simulink model "GVCU_HIL"  (R2026a)
settings: Solver=ode3  StartTime=0  StopTime=2474  FixedStep=0.0002
model workspace (MAT data in the model file):
  CANoelibParameters : object (value not decoded)
values from neighbouring files (symbols this model uses):
  acc_pedal_data = pedal_data.accelerator_pedal_position_t0    [Vehicle_Simulink_init.m]
  acc_pedal_time = pedal_data.t0    [Vehicle_Simulink_init.m]
  brk_pedal_data = brake_pedal_data.shared_brakes_drvrBrkPedlPerc_t0    [Vehicle_Simulink_init.m]
  brk_pedal_time = brake_pedal_data.t0    [Vehicle_Simulink_init.m]
  cycle_len = zeros(1, num_cycles)    [Vehicle_Simulink_init.m]
  cycle_speed_matrix = zeros(max_cycle_len, num_cycles)    [Vehicle_Simulink_init.m]
  cycle_time_matrix = zeros(max_cycle_len, num_cycles)    [Vehicle_Simulink_init.m]
  veh_speed_data = speed_data.shared_dynamicsVso_vehVelLgt_t0    [Vehicle_Simulink_init.m]
  veh_speed_time = speed_data.t0    [Vehicle_Simulink_init.m]
undefined symbols (not defined in the file or in its folder): Active, AuxActive, bat, environment, FL_prs_voltage, FR_prs_voltage, pos, RL_prs_voltage, RR_prs_voltage, tir, veh, VGetRawValueFlag, Voltage, VT2816_1_Ch1, VT2816_1_Ch2, VT2816_1_Ch3, VT2816_1_Ch4, VT2816_3_Ch13, VT2816_3_Ch14, VT7101_1_Out2, VT7820_2_Channel1, VT7820_2_Channel2, VT7820_2_Channel3, VT7820_2_Channel4, VTS
libraries: canoelib x144, autolibsharedcoupling x21, autolibcoupling x9, autolibshared x5, simulink_extras x4, simulink x4, slpidlib x3, autolibshareddiff x3, autolibutils x1, autolibdatasheetbattery x1, autolibmappedmotor x1, sl_discontinuities x1
(part 4 of 9)

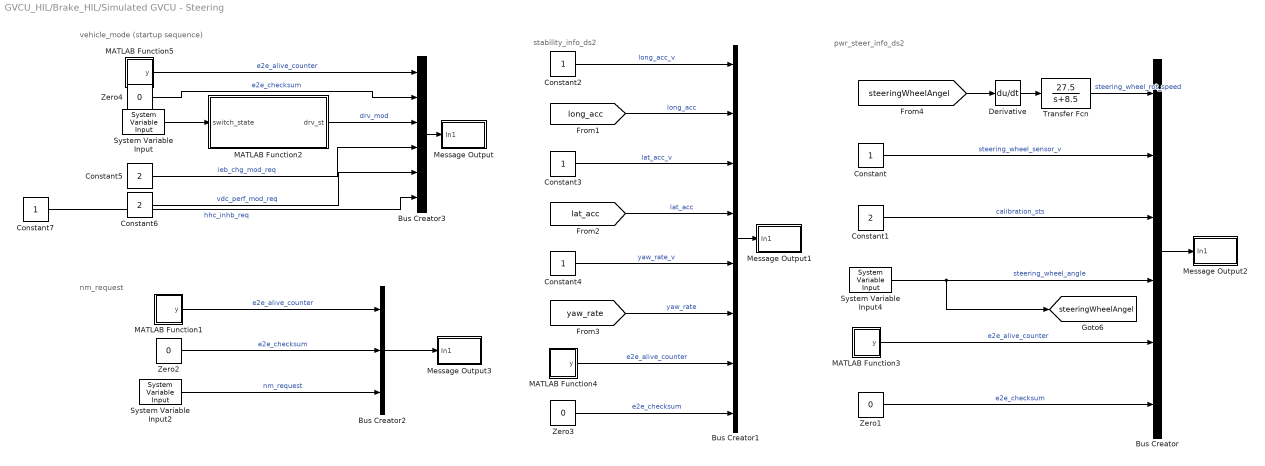
== system GVCU_HIL/Brake_HIL/Simulated GVCU - Steering  ==
  note: pwr_steer_info_ds2
  note: stability_info_ds2
  note: vehicle_mode (startup sequence)
  note: nm_request
  Bus Creator : BusCreator  Inputs=6
  Bus Creator1 : BusCreator  Inputs=8
  Bus Creator2 : BusCreator  Inputs=3
  Bus Creator3 : BusCreator  Inputs=6
  Constant{,2..4,7} (5 alike) : Constant
  Constant1 : Constant  Value=2
  Constant5 : Constant  Value=2
  Constant6 : Constant  Value=2
  Derivative : Derivative
  MATLAB Function1 : MATLAB Function  TreatAsAtomicUnit=on
  MATLAB Function2 : MATLAB Function  TreatAsAtomicUnit=on
  MATLAB Function3 : MATLAB Function  TreatAsAtomicUnit=on
  MATLAB Function4 : MATLAB Function  TreatAsAtomicUnit=on
  MATLAB Function5 : MATLAB Function  TreatAsAtomicUnit=on
  Message Output : Subsystem  AncestorBlock=canoelib/CANoe I//O/Message Output  mask(Signal Output Module){dbName=IEB_DBC_V32, nodeName=GVCU, msgName=vehicle_mode, inputType=Bus Signal, rawValue=Default}
      mask prompts: dbName "Database name"; nodeName "Node name"; msgName "Message name"; inputType "Input type"; rawValue "Raw value"
      mask help: Output module for all signals of a databasemessage provided by the CANoe interaction layer. Double click the block for configuration.
      settings: AttributesFormatString=%<msgName>  CopyFcn=set_param(gcb, 'AttributesFormatString', '%<msgName>');  OpenFcn=MessageOutputBlock
      mask Help: For detailed information please refer to the CANoe online help 'MATLAB Integration Package » CANoe I/O Library'.
      mask TypeOptions inputType: Vector | Bus Signal
      mask TypeOptions rawValue: Default | Physical value | Raw value
      mask Display:
      | image(imread('MatlabBlock.png'))
      | disp('CANoe')
  Message Output1 : Subsystem  AncestorBlock=canoelib/CANoe I//O/Message Output  mask(Signal Output Module){dbName=IEB_DBC_V32, nodeName=GVCU, msgName=stability_info_ds2, inputType=Bus Signal, rawValue=Default}
      mask prompts: dbName "Database name"; nodeName "Node name"; msgName "Message name"; inputType "Input type"; rawValue "Raw value"
      mask help: Output module for all signals of a databasemessage provided by the CANoe interaction layer. Double click the block for configuration.
      settings: AttributesFormatString=%<msgName>  CopyFcn=set_param(gcb, 'AttributesFormatString', '%<msgName>');  OpenFcn=MessageOutputBlock
      mask Help: For detailed information please refer to the CANoe online help 'MATLAB Integration Package » CANoe I/O Library'.
      mask TypeOptions inputType: Vector | Bus Signal
      mask TypeOptions rawValue: Default | Physical value | Raw value
      mask Display:
      | image(imread('MatlabBlock.png'))
      | disp('CANoe')
  Message Output2 : Subsystem  AncestorBlock=canoelib/CANoe I//O/Message Output  mask(Signal Output Module){dbName=IEB_DBC_V32, nodeName=GVCU, msgName=pwr_steer_info_ds2, inputType=Bus Signal, rawValue=Default}
      mask prompts: dbName "Database name"; nodeName "Node name"; msgName "Message name"; inputType "Input type"; rawValue "Raw value"
      mask help: Output module for all signals of a databasemessage provided by the CANoe interaction layer. Double click the block for configuration.
      settings: AttributesFormatString=%<msgName>  CopyFcn=set_param(gcb, 'AttributesFormatString', '%<msgName>');  OpenFcn=MessageOutputBlock
      mask Help: For detailed information please refer to the CANoe online help 'MATLAB Integration Package » CANoe I/O Library'.
      mask TypeOptions inputType: Vector | Bus Signal
      mask TypeOptions rawValue: Default | Physical value | Raw value
      mask Display:
      | image(imread('MatlabBlock.png'))
      | disp('CANoe')
  Message Output3 : Subsystem  AncestorBlock=canoelib/CANoe I//O/Message Output  mask(Signal Output Module){dbName=IEB_DBC_V32, nodeName=GVCU, msgName=nm_request_gvcu_ds2, inputType=Bus Signal, rawValue=Default}
      mask prompts: dbName "Database name"; nodeName "Node name"; msgName "Message name"; inputType "Input type"; rawValue "Raw value"
      mask help: Output module for all signals of a databasemessage provided by the CANoe interaction layer. Double click the block for configuration.
      settings: AttributesFormatString=%<msgName>  CopyFcn=set_param(gcb, 'AttributesFormatString', '%<msgName>');  OpenFcn=MessageOutputBlock
      mask Help: For detailed information please refer to the CANoe online help 'MATLAB Integration Package » CANoe I/O Library'.
      mask TypeOptions inputType: Vector | Bus Signal
      mask TypeOptions rawValue: Default | Physical value | Raw value
      mask Display:
      | image(imread('MatlabBlock.png'))
      | disp('CANoe')
  System Variable Input : canoelib/CANoe I//O/System Variable Input  nsName=ABS_TEST  sysVarName=Acceleration  arrayIndex=-1  editSampleTime=0  rawValue=Default  dataType=Default  dataTypeDB=int32  hasEncoding=off  dataTypeCANoe=Get from CANoe
      settings: AttributesFormatString=%<nsName>::%<sysVarName>  SourceProductName=Vector CANoe
  System Variable Input2 : canoelib/CANoe I//O/System Variable Input  nsName=ABS_TEST  sysVarName=NM_request_Model  arrayIndex=-1  editSampleTime=0  rawValue=Default  dataType=Default  dataTypeDB=uint32  hasEncoding=off  dataTypeCANoe=Get from CANoe
      settings: AttributesFormatString=%<nsName>::%<sysVarName>  SourceProductName=Vector CANoe
  System Variable Input4 : canoelib/CANoe I//O/System Variable Input  nsName=ABS_TEST  sysVarName=steering_ang  arrayIndex=-1  editSampleTime=0  rawValue=Default  dataType=Default  dataTypeDB=double  hasEncoding=off  dataTypeCANoe=Get from CANoe
      settings: AttributesFormatString=%<nsName>::%<sysVarName>  SourceProductName=Vector CANoe
  Transfer Fcn : TransferFcn  Numerator=[27.5]  Denominator=[1 8.5]
  Zero{1..4} (4 alike) : Constant  Value=0  OutDataTypeStr=Inherit: Inherit via back propagation
  tag scope: steeringWheelAngel=global
  wires:
  Transfer Fcn/1 -> Bus Creator/1  "steering_wheel_rot_speed"
  Derivative/1 -> Transfer Fcn/1
  [steeringWheelAngel] -> Derivative/1
  MATLAB Function1/1(y) -> Bus Creator2/1  "e2e_alive_counter"
  MATLAB Function4/1(y) -> Bus Creator1/7  "e2e_alive_counter"
  MATLAB Function5/1(y) -> Bus Creator3/1  "e2e_alive_counter"
  MATLAB Function3/1(y) -> Bus Creator/5  "e2e_alive_counter"
  Bus Creator3/1 -> Message Output/1(In1)
  Zero4/1 -> Bus Creator3/2  "e2e_checksum"
  Bus Creator2/1 -> Message Output3/1(In1)
  Zero2/1 -> Bus Creator2/2  "e2e_checksum"
  System Variable Input2/1 -> Bus Creator2/3  "nm_request"
  Constant6/1 -> Bus Creator3/5  "vdc_perf_mod_req"
  Constant5/1 -> Bus Creator3/4  "ieb_chg_mod_req"
  System Variable Input/1 -> MATLAB Function2/1(switch_state)
  MATLAB Function2/1(drv_st) -> Bus Creator3/3  "drv_mod"
  Bus Creator1/1 -> Message Output1/1(In1)
  [yaw_rate] -> Bus Creator1/6  "yaw_rate"
  [long_acc] -> Bus Creator1/2  "long_acc"
  [lat_acc] -> Bus Creator1/4  "lat_acc"
  Zero3/1 -> Bus Creator1/8  "e2e_checksum"
  Constant4/1 -> Bus Creator1/5  "yaw_rate_v"
  Constant3/1 -> Bus Creator1/3  "lat_acc_v"
  Constant2/1 -> Bus Creator1/1  "long_acc_v"
  Bus Creator/1 -> Message Output2/1(In1)
  Zero1/1 -> Bus Creator/6  "e2e_checksum"
  System Variable Input4/1 -> Bus Creator/4, [steeringWheelAngel]  "steering_wheel_angle"
  Constant1/1 -> Bus Creator/3  "calibration_sts"
  Constant7/1 -> Bus Creator3/6  "hhc_inhb_req"
  Constant/1 -> Bus Creator/2  "steering_wheel_sensor_v"

== system GVCU_HIL/Clutch handling/Offset prs setting ==
  prs_to_voltage : Inport
  Offset setting : Constant  Value=0
  Step : Step  Time=0.2  SampleTime=0
  Switch : Switch  Criteria=u2 > Threshold  SaturateOnIntegerOverflow=off  InputSameDT=off
  Out1 : Outport
  wires:
  Step/1 -> Switch/2
  Offset setting/1 -> Switch/3
  Switch/1 -> Out1/1
  prs_to_voltage/1 -> Switch/1

== system GVCU_HIL/Clutch handling/Offset prs setting1 ==
  prs_to_voltage : Inport
  Offset setting : Constant  Value=0
  Step : Step  Time=0.2  SampleTime=0
  Switch : Switch  Criteria=u2 > Threshold  SaturateOnIntegerOverflow=off  InputSameDT=off
  Out1 : Outport
  wires:
  Step/1 -> Switch/2
  Offset setting/1 -> Switch/3
  Switch/1 -> Out1/1
  prs_to_voltage/1 -> Switch/1

== system GVCU_HIL/Clutch handling/Offset prs setting2 ==
  prs_to_voltage : Inport
  Offset setting : Constant  Value=0
  Step : Step  Time=0.2  SampleTime=0
  Switch : Switch  Criteria=u2 > Threshold  SaturateOnIntegerOverflow=off  InputSameDT=off
  Out1 : Outport
  wires:
  Step/1 -> Switch/2
  Offset setting/1 -> Switch/3
  Switch/1 -> Out1/1
  prs_to_voltage/1 -> Switch/1

== system GVCU_HIL/Clutch handling/Offset prs setting3 ==
  prs_to_voltage : Inport
  Offset setting : Constant  Value=0
  Step : Step  Time=0.2  SampleTime=0
  Switch : Switch  Criteria=u2 > Threshold  SaturateOnIntegerOverflow=off  InputSameDT=off
  Out1 : Outport
  wires:
  Step/1 -> Switch/2
  Offset setting/1 -> Switch/3
  Switch/1 -> Out1/1
  prs_to_voltage/1 -> Switch/1

== system GVCU_HIL/Clutch handling/Offset_substraction ==
  prs_to_voltage : Inport
  MATLAB Function : MATLAB Function  TreatAsAtomicUnit=on
  Signal Input : canoelib/CANoe I//O/Signal Input  dbName=dynamic_systems1_bus  nodeName=GVCU  msgName=vehicle_status_ds1  sigName=drv_mod  editSampleTime=0  rawValue=Default  dataType=Default  dataTypeDB=uint8  hasEncoding=off
      settings: AttributesFormatString=%<sigName>  SourceProductName=Vector CANoe
  y : Outport
  wires:
  Signal Input/1 -> MATLAB Function/1(drvMode)
  MATLAB Function/1(y) -> y/1
  prs_to_voltage/1 -> MATLAB Function/2(pPa)

== system GVCU_HIL/Clutch handling/cur_to_prs ==
  note: Dither filtering
  note: breakpoints out of real measurement
  In1 : Inport
  1-D Lookup Table2 : Lookup_n-D  NumberOfTableDimensions=1  BreakpointsForDimension1=[14.52 16.75 17.32 24.99]  Table=[1.02 3.38 3.68 11.09]  InternalRulePriority=Speed  RndMeth=Simplest
  1-D Lookup Table9 : Lookup_n-D  NumberOfTableDimensions=1  BreakpointsForDimension1=[0.584 0.786 0.882 0.992]  Table=[14.62 19.62 22.19 24.95]  InternalRulePriority=Speed  RndMeth=Simplest
  Constant : Constant  Value=0
  Gain : Gain  Gain=100000
  Switch2 : Switch  Criteria=u2 > Threshold  Threshold=0.1  SaturateOnIntegerOverflow=off  InputSameDT=off
  Transfer Fcn : TransferFcn  Denominator=[1 1]
  Out1 : Outport
  wires:
  Switch2/1 -> Out1/1
  1-D Lookup Table9/1 -> 1-D Lookup Table2/1  "cluCMD [%]"
  In1/1 -> Transfer Fcn/1  "solnDrvrCur [A]"
  Constant/1 -> Switch2/3
  1-D Lookup Table2/1 -> Gain/1  "whlCluPress [bar]"
  Gain/1 -> Switch2/1  "[Pa]"
  Transfer Fcn/1 -> 1-D Lookup Table9/1, Switch2/2

== system GVCU_HIL/Clutch handling/cur_to_prs1 ==
  note: Dither filtering
  note: breakpoints out of real measurement
  In1 : Inport
  1-D Lookup Table2 : Lookup_n-D  NumberOfTableDimensions=1  BreakpointsForDimension1=[14.52 16.75 17.32 24.99]  Table=[1.02 3.38 3.68 11.09]  InternalRulePriority=Speed  RndMeth=Simplest
  1-D Lookup Table9 : Lookup_n-D  NumberOfTableDimensions=1  BreakpointsForDimension1=[0.584 0.786 0.882 0.992]  Table=[14.62 19.62 22.19 24.95]  InternalRulePriority=Speed  RndMeth=Simplest
  Constant : Constant  Value=0
  Gain : Gain  Gain=100000
  Switch2 : Switch  Criteria=u2 > Threshold  Threshold=0.1  SaturateOnIntegerOverflow=off  InputSameDT=off
  Transfer Fcn : TransferFcn  Denominator=[1 1]
  Out1 : Outport
  wires:
  Switch2/1 -> Out1/1
  1-D Lookup Table9/1 -> 1-D Lookup Table2/1  "cluCMD [%]"
  In1/1 -> Transfer Fcn/1  "solnDrvrCur [A]"
  Constant/1 -> Switch2/3
  1-D Lookup Table2/1 -> Gain/1  "whlCluPress [bar]"
  Gain/1 -> Switch2/1  "[Pa]"
  Transfer Fcn/1 -> 1-D Lookup Table9/1, Switch2/2

== system GVCU_HIL/Clutch handling/cur_to_prs2 ==
  note: Dither filtering
  note: breakpoints out of real measurement
  In1 : Inport
  1-D Lookup Table2 : Lookup_n-D  NumberOfTableDimensions=1  BreakpointsForDimension1=[14.52 16.75 17.32 24.99]  Table=[1.02 3.38 3.68 11.09]  InternalRulePriority=Speed  RndMeth=Simplest
  1-D Lookup Table9 : Lookup_n-D  NumberOfTableDimensions=1  BreakpointsForDimension1=[0.584 0.786 0.882 0.992]  Table=[14.62 19.62 22.19 24.95]  InternalRulePriority=Speed  RndMeth=Simplest
  Constant : Constant  Value=0
  Gain : Gain  Gain=100000
  Switch2 : Switch  Criteria=u2 > Threshold  Threshold=0.1  SaturateOnIntegerOverflow=off  InputSameDT=off
  Transfer Fcn : TransferFcn  Denominator=[1 1]
  Out1 : Outport
  wires:
  Switch2/1 -> Out1/1
  1-D Lookup Table9/1 -> 1-D Lookup Table2/1  "cluCMD [%]"
  In1/1 -> Transfer Fcn/1  "solnDrvrCur [A]"
  Constant/1 -> Switch2/3
  1-D Lookup Table2/1 -> Gain/1  "whlCluPress [bar]"
  Gain/1 -> Switch2/1  "[Pa]"
  Transfer Fcn/1 -> 1-D Lookup Table9/1, Switch2/2

== system GVCU_HIL/Clutch handling/cur_to_prs3 ==
  note: Dither filtering
  note: breakpoints out of real measurement
  In1 : Inport
  1-D Lookup Table2 : Lookup_n-D  NumberOfTableDimensions=1  BreakpointsForDimension1=[14.52 16.75 17.32 24.99]  Table=[1.02 3.38 3.68 11.09]  InternalRulePriority=Speed  RndMeth=Simplest
  1-D Lookup Table9 : Lookup_n-D  NumberOfTableDimensions=1  BreakpointsForDimension1=[0.584 0.786 0.882 0.992]  Table=[14.62 19.62 22.19 24.95]  InternalRulePriority=Speed  RndMeth=Simplest
  Constant : Constant  Value=0
  Gain : Gain  Gain=100000
  Switch2 : Switch  Criteria=u2 > Threshold  Threshold=0.1  SaturateOnIntegerOverflow=off  InputSameDT=off
  Transfer Fcn : TransferFcn  Denominator=[1 1]
  Out1 : Outport
  wires:
  Switch2/1 -> Out1/1
  1-D Lookup Table9/1 -> 1-D Lookup Table2/1  "cluCMD [%]"
  In1/1 -> Transfer Fcn/1  "solnDrvrCur [A]"
  Constant/1 -> Switch2/3
  1-D Lookup Table2/1 -> Gain/1  "whlCluPress [bar]"
  Gain/1 -> Switch2/1  "[Pa]"
  Transfer Fcn/1 -> 1-D Lookup Table9/1, Switch2/2

== system GVCU_HIL/Driver/Driver ==
  Vel_ref : Inport
  Vel_fdbk : Inport  Port=2
  Dec_panel 0 -100 : Inport  Port=3
  "0 to 1 " : Saturate  UpperLimit=1  LowerLimit=0
  Compare To Constant : simulink/Logic and Bit Operations/Compare To Constant  relop=>  const=0  OutDataTypeStr=boolean
  Constant : Constant  Value=0
  Constant1 : Constant  Value=0
  Dec_controller : Subsystem
  Gain : Gain  Gain=100
  Integrator1 : Integrator  ExternalReset=level  LimitOutput=on  UpperSaturationLimit=1  LowerSaturationLimit=-1
  Kaw : Gain  SaturateOnIntegerOverflow=on  OutDataTypeStr=Inherit: Same as input  ParamDataTypeStr=Inherit: Same as input
  Kff : Gain  Gain=0.005  SaturateOnIntegerOverflow=on  OutDataTypeStr=Inherit: Same as input  ParamDataTypeStr=Inherit: Same as input
  Ki : Gain  Gain=0.0286  SaturateOnIntegerOverflow=on  OutDataTypeStr=Inherit: Same as input  ParamDataTypeStr=Inherit: Same as input
  LPF : Subsystem
  Subtract : Sum  Inputs=+-
  Subtract1 : Sum  Inputs=-+
  Sum1 : Sum  Inputs=+++  InputSameDT=on  SaturateOnIntegerOverflow=on  OutDataTypeStr=Inherit: Same as first input
  Sum8 : Sum  InputSameDT=on  SaturateOnIntegerOverflow=on  OutDataTypeStr=Inherit: Same as first input
  Switch{,1..3} (4 alike) : Switch  Criteria=u2 > Threshold  SaturateOnIntegerOverflow=off  InputSameDT=off
  System Variable Output : canoelib/CANoe I//O/System Variable Output  nsName=Checker_Simulink  sysVarName=Test_param  arrayIndex=-1  rawValue=Default  dataType=Default  dataTypeDB=int32  hasEncoding=off  dataTypeCANoe=Get from CANoe
      settings: AttributesFormatString=%<nsName>::%<sysVarName>  SourceProductName=Vector CANoe
  kp : Gain  Gain=0.286  SaturateOnIntegerOverflow=on  OutDataTypeStr=Inherit: Same as input  ParamDataTypeStr=Inherit: Same as input
  acc_cmd : Outport
  dec_cmd : Outport  Port=2
  wires:
  Kaw/1 -> Sum8/2
  Integrator1/1 -> Sum1/3
  Kff/1 -> Sum1/1
  Sum8/1 -> Integrator1/1
  Sum1/1 -> Subtract1/1, "0 to 1 "/1
  kp/1 -> Sum1/2
  Switch1/1 -> Subtract/1, Kff/1
  Ki/1 -> Sum8/1
  Subtract/1 -> LPF/1(u)  "error"
  LPF/1(y) -> kp/1, Ki/1
  Switch/1 -> dec_cmd/1
  Constant/1 -> Switch/3
  "0 to 1 "/1 -> Subtract1/2, Gain/1
  Gain/1 -> acc_cmd/1  "AccelCmd"
  Switch3/1 -> Compare To Constant/1, Switch/1, System Variable Output/1, Switch/2, Switch2/2, Switch1/2
  Subtract1/1 -> Switch2/3
  Vel_ref/1 -> Dec_controller/1(Vel_ref), Switch1/3
  Compare To Constant/1 -> Integrator1/2
  Switch2/1 -> Kaw/1
  Constant1/1 -> Switch2/1
  Dec_panel 0 -100/1 -> Switch3/2, Switch3/1
  Dec_controller/1(Dec_cmd) -> Switch3/3
  Vel_fdbk/1 -> Dec_controller/2(Vel_fdk), Switch1/1, Subtract/2

== system GVCU_HIL/Driver/Subsystem ==
  Enable : EnablePort
  Drive Cycle Source : autolibshared/Drive Cycle Source  cycleVar=FTP75  fileVar=cycleFTP75.mat  tfinal="2474  seconds"  cycleRepeat=off  outAccPort=off  outGearPort=off  gearList=No gear data  t_wot1=5  xdot_woto=0  xdot_wot1=30  t_wot2=20  xdot_wot2=0  t_wotend=30  srcUnit=m/s  outUnit=m/s  srcAccUnit=m/s/s  outAccUnit=m/s^2  dt=0  aMode=1  faultOption=off  velBnd=2  velBndUnit=mph  inUnit=m/s  timeBnd=1  failOption=off  stopSim=off  maxFaultCnt=10  maxFaultTime=2  maxTotFaultTime=15  traceOption=off  dtTrace=1  traceWindow=10  lastDCname=FTP75  lastOutUnit=mph  lastDT=0  lastTB=1  lastSB=2  forceCalcBound=off
      link override Timing Mode: LabelModeActiveChoice=1
      link override Timing Mode/Continuous/FaultSystem/Fault Mode: LabelModeActiveChoice=1
      link override Timing Mode/Continuous/FaultSystem/Fault Mode/Fault On/FailureBlock: LabelModeActiveChoice=1
      link override Timing Mode/Continuous/FaultSystem/TracePlot: LabelModeActiveChoice=1
      link override Timing Mode/Discrete/FaultSystem/Fault Mode: LabelModeActiveChoice=1
      link override Timing Mode/Discrete/FaultSystem/Fault Mode/Fault On/FailureBlock: LabelModeActiveChoice=1
      link override Timing Mode/Discrete/FaultSystem/TracePlot: LabelModeActiveChoice=1
  drive_cycle_speed : Outport
  wires:
  Drive Cycle Source/1 -> drive_cycle_speed/1  "m/s"

== system GVCU_HIL/Environment/Air ==
  Bus Creator : BusCreator  Inputs=3
  Constant : Constant  Value=environment.air.temp
  Constant1 : Constant  Value=environment.air.prs
  Constant2 : Constant  Value=environment.air.density
  Air : Outport  VectorParamsAs1DForOutWhenUnconnected=off
  wires:
  Constant/1 -> Bus Creator/1  "temprature"
  Bus Creator/1 -> Air/1
  Constant1/1 -> Bus Creator/2  "pressure"
  Constant2/1 -> Bus Creator/3  "density"

== system GVCU_HIL/Environment/Friction ==
  Bus Creator : BusCreator  Inputs=2
  Constant : Constant  Value=environment.mu.x
  Constant1 : Constant  Value=environment.mu.y
  Friction : Outport  VectorParamsAs1DForOutWhenUnconnected=off
  wires:
  Bus Creator/1 -> Friction/1
  Constant/1 -> Bus Creator/1  "mux"
  Constant1/1 -> Bus Creator/2  "muy"

== system GVCU_HIL/Environment/Ground ==
  Bus Creator2 : BusCreator  Inputs=5
  Constant{,1..3} (4 alike) : Constant  Value=0
  DCM : Constant  Value=repmat(eye(3),1,1,4)
  Ground : Outport
  wires:
  Bus Creator2/1 -> Ground/1  "z"
  Constant/1 -> Bus Creator2/1  "G_FL_z"
  DCM/1 -> Bus Creator2/5  "DCM"
  Constant1/1 -> Bus Creator2/2  "G_FR_z"
  Constant3/1 -> Bus Creator2/4  "G_RR_z"
  Constant2/1 -> Bus Creator2/3  "G_RL_z"

== system GVCU_HIL/Environment/Wind ==
  Bus Creator : BusCreator  Inputs=3
  wind x : Constant  Value=environment.wind.x
  wind y : Constant  Value=environment.wind.y
  wind z : Constant  Value=environment.wind.z
  Wind : Outport  VectorParamsAs1DForOutWhenUnconnected=off
  wires:
  Bus Creator/1 -> Wind/1
  wind x/1 -> Bus Creator/1  "windx"
  wind y/1 -> Bus Creator/2  "windy"
  wind z/1 -> Bus Creator/3  "windz"

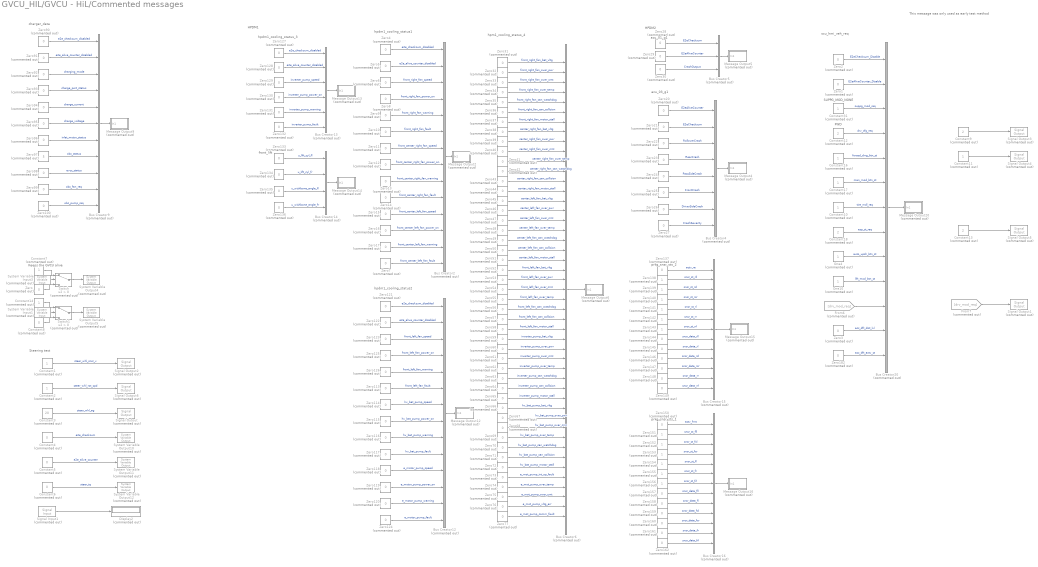
== system GVCU_HIL/GVCU - HiL/Commented messages ==
  note: HPDM2
  note: prkg_snsr_sts_2
  note: front_lift
  note: HPDM1
  note: hpdm1_cooling_status_3
  note: hpm1_cooling_status_4
  note: acu_01_g1
  note: acu_03_g1
  note: hpdm1_cooling_status1
  note: hpdm1_cooling_status2
  note: prkg_snsr_sts_1
  note: FWD
  note: This message was only used as early test method
  note: SUPPG_MOD_NONE
  note: scu_hmi_veh_req
  note: charger_data
  note: Steering test
  note: Keeps the GVCU alive
  Bus Creator12 : BusCreator  Commented=on  Inputs=14
  Bus Creator13 : BusCreator  Commented=on  Inputs=6
  Bus Creator14 : BusCreator  Commented=on  Inputs=4
  Bus Creator15 : BusCreator  Commented=on  Inputs=13
  Bus Creator16 : BusCreator  Commented=on  Inputs=13
  Bus Creator2 : BusCreator  Commented=on  Inputs=14
  Bus Creator20 : BusCreator  Commented=on  Inputs=13
  Bus Creator4 : BusCreator  Commented=on  Inputs=8
  Bus Creator5 : BusCreator  Commented=on  Inputs=3
  Bus Creator6 : BusCreator  Commented=on  Inputs=47
  Bus Creator9 : BusCreator  Commented=on  Inputs=11
  Constant{1..2,7,10..11,14,16..17,31} (9 alike) : Constant  Commented=on
  Constant{9,12..13,18} (4 alike) : Constant  Commented=on  Value=2
  Constant3 : Constant  Commented=on  Value=20
  Constant4 : Constant  Commented=on  Value=0  OutMin=0  OutMax=15  OutDataTypeStr=int32
  Constant5 : Constant  Commented=on  Value=0  OutMin=0  OutMax=15  OutDataTypeStr=int32
  Constant6 : Constant  Commented=on  Value=0
  Constant8 : Constant  Commented=on  Value=0
  Display2 : Display  Commented=on
  From6 : From  Commented=on  GotoTag=drv_mod_req  TagVisibility=global
  From7 : From  Commented=on  GotoTag=drv_mod_req  TagVisibility=global
  Message Output12 : Subsystem  Commented=on  AncestorBlock=canoelib/CANoe I//O/Message Output  mask(Signal Output Module){dbName=main_bus, nodeName=HPDM1, msgName=hpdm1_cooling_status2, inputType=Bus Signal, rawValue=Default}
      mask prompts: dbName "Database name"; nodeName "Node name"; msgName "Message name"; inputType "Input type"; rawValue "Raw value"
      mask help: Output module for all signals of a databasemessage provided by the CANoe interaction layer. Double click the block for configuration.
      settings: AttributesFormatString=%<msgName>  CopyFcn=set_param(gcb, 'AttributesFormatString', '%<msgName>');  OpenFcn=MessageOutputBlock
      mask Help: For detailed information please refer to the CANoe online help 'MATLAB Integration Package » CANoe I/O Library'.
      mask TypeOptions inputType: Vector | Bus Signal
      mask TypeOptions rawValue: Default | Physical value | Raw value
      mask Display:
      | image(imread('MatlabBlock.png'))
      | disp('CANoe')
  Message Output13 : Subsystem  Commented=on  AncestorBlock=canoelib/CANoe I//O/Message Output  mask(Signal Output Module){dbName=main_bus, nodeName=HPDM1, msgName=hpdm1_cooling_status3, inputType=Bus Signal, rawValue=Default}
      mask prompts: dbName "Database name"; nodeName "Node name"; msgName "Message name"; inputType "Input type"; rawValue "Raw value"
      mask help: Output module for all signals of a databasemessage provided by the CANoe interaction layer. Double click the block for configuration.
      settings: AttributesFormatString=%<msgName>  CopyFcn=set_param(gcb, 'AttributesFormatString', '%<msgName>');  OpenFcn=MessageOutputBlock
      mask Help: For detailed information please refer to the CANoe online help 'MATLAB Integration Package » CANoe I/O Library'.
      mask TypeOptions inputType: Vector | Bus Signal
      mask TypeOptions rawValue: Default | Physical value | Raw value
      mask Display:
      | image(imread('MatlabBlock.png'))
      | disp('CANoe')
  Message Output14 : Subsystem  Commented=on  AncestorBlock=canoelib/CANoe I//O/Message Output  mask(Signal Output Module){dbName=main_bus, nodeName=HPDM1, msgName=front_lift_status, inputType=Bus Signal, rawValue=Default}
      mask prompts: dbName "Database name"; nodeName "Node name"; msgName "Message name"; inputType "Input type"; rawValue "Raw value"
      mask help: Output module for all signals of a databasemessage provided by the CANoe interaction layer. Double click the block for configuration.
      settings: AttributesFormatString=%<msgName>  CopyFcn=set_param(gcb, 'AttributesFormatString', '%<msgName>');  OpenFcn=MessageOutputBlock
      mask Help: For detailed information please refer to the CANoe online help 'MATLAB Integration Package » CANoe I/O Library'.
      mask TypeOptions inputType: Vector | Bus Signal
      mask TypeOptions rawValue: Default | Physical value | Raw value
      mask Display:
      | image(imread('MatlabBlock.png'))
      | disp('CANoe')
  Message Output15 : Subsystem  Commented=on  AncestorBlock=canoelib/CANoe I//O/Message Output  mask(Signal Output Module){dbName=main_bus, nodeName=HPDM2, msgName=prkg_snsr_st_2, inputType=Bus Signal, rawValue=Default}
      mask prompts: dbName "Database name"; nodeName "Node name"; msgName "Message name"; inputType "Input type"; rawValue "Raw value"
      mask help: Output module for all signals of a databasemessage provided by the CANoe interaction layer. Double click the block for configuration.
      settings: AttributesFormatString=%<msgName>  CopyFcn=set_param(gcb, 'AttributesFormatString', '%<msgName>');  OpenFcn=MessageOutputBlock
      mask Help: For detailed information please refer to the CANoe online help 'MATLAB Integration Package » CANoe I/O Library'.
      mask TypeOptions inputType: Vector | Bus Signal
      mask TypeOptions rawValue: Default | Physical value | Raw value
      mask Display:
      | image(imread('MatlabBlock.png'))
      | disp('CANoe')
  Message Output16 : Subsystem  Commented=on  AncestorBlock=canoelib/CANoe I//O/Message Output  mask(Signal Output Module){dbName=main_bus, nodeName=HPDM2, msgName=prkg_snsr_st_1, inputType=Bus Signal, rawValue=Default}
      mask prompts: dbName "Database name"; nodeName "Node name"; msgName "Message name"; inputType "Input type"; rawValue "Raw value"
      mask help: Output module for all signals of a databasemessage provided by the CANoe interaction layer. Double click the block for configuration.
      settings: AttributesFormatString=%<msgName>  CopyFcn=set_param(gcb, 'AttributesFormatString', '%<msgName>');  OpenFcn=MessageOutputBlock
      mask Help: For detailed information please refer to the CANoe online help 'MATLAB Integration Package » CANoe I/O Library'.
      mask TypeOptions inputType: Vector | Bus Signal
      mask TypeOptions rawValue: Default | Physical value | Raw value
      mask Display:
      | image(imread('MatlabBlock.png'))
      | disp('CANoe')
  Message Output2 : Subsystem  Commented=on  AncestorBlock=canoelib/CANoe I//O/Message Output  mask(Signal Output Module){dbName=main_bus, nodeName=HPDM1, msgName=hpdm1_cooling_status1, inputType=Bus Signal, rawValue=Default}
      mask prompts: dbName "Database name"; nodeName "Node name"; msgName "Message name"; inputType "Input type"; rawValue "Raw value"
      mask help: Output module for all signals of a databasemessage provided by the CANoe interaction layer. Double click the block for configuration.
      settings: AttributesFormatString=%<msgName>  CopyFcn=set_param(gcb, 'AttributesFormatString', '%<msgName>');  OpenFcn=MessageOutputBlock
      mask Help: For detailed information please refer to the CANoe online help 'MATLAB Integration Package » CANoe I/O Library'.
      mask TypeOptions inputType: Vector | Bus Signal
      mask TypeOptions rawValue: Default | Physical value | Raw value
      mask Display:
      | image(imread('MatlabBlock.png'))
      | disp('CANoe')
  Message Output20 : Subsystem  Commented=on  AncestorBlock=canoelib/CANoe I//O/Message Output  mask(Signal Output Module){dbName=main_bus, nodeName=SCU, msgName=scu_hmi_veh_req, inputType=Bus Signal, rawValue=Default}
      mask prompts: dbName "Database name"; nodeName "Node name"; msgName "Message name"; inputType "Input type"; rawValue "Raw value"
      mask help: Output module for all signals of a databasemessage provided by the CANoe interaction layer. Double click the block for configuration.
      settings: AttributesFormatString=%<msgName>  CopyFcn=set_param(gcb, 'AttributesFormatString', '%<msgName>');  OpenFcn=MessageOutputBlock
      mask Help: For detailed information please refer to the CANoe online help 'MATLAB Integration Package » CANoe I/O Library'.
      mask TypeOptions inputType: Vector | Bus Signal
      mask TypeOptions rawValue: Default | Physical value | Raw value
      mask Display:
      | image(imread('MatlabBlock.png'))
      | disp('CANoe')
  Message Output4 : Subsystem  Commented=on  AncestorBlock=canoelib/CANoe I//O/Message Output  mask(Signal Output Module){dbName=inverter_bus, nodeName=GVCU, msgName=acu_03_g2, inputType=Bus Signal, rawValue=Default}
      mask prompts: dbName "Database name"; nodeName "Node name"; msgName "Message name"; inputType "Input type"; rawValue "Raw value"
      mask help: Output module for all signals of a databasemessage provided by the CANoe interaction layer. Double click the block for configuration.
      settings: AttributesFormatString=%<msgName>  CopyFcn=set_param(gcb, 'AttributesFormatString', '%<msgName>');  OpenFcn=MessageOutputBlock
      mask Help: For detailed information please refer to the CANoe online help 'MATLAB Integration Package » CANoe I/O Library'.
      mask TypeOptions inputType: Vector | Bus Signal
      mask TypeOptions rawValue: Default | Physical value | Raw value
      mask Display:
      | image(imread('MatlabBlock.png'))
      | disp('CANoe')
  Message Output5 : Subsystem  Commented=on  AncestorBlock=canoelib/CANoe I//O/Message Output  mask(Signal Output Module){dbName=main_bus, nodeName=HPDM2, msgName=acu_01_g1, inputType=Bus Signal, rawValue=Default}
      mask prompts: dbName "Database name"; nodeName "Node name"; msgName "Message name"; inputType "Input type"; rawValue "Raw value"
      mask help: Output module for all signals of a databasemessage provided by the CANoe interaction layer. Double click the block for configuration.
      settings: AttributesFormatString=%<msgName>  CopyFcn=set_param(gcb, 'AttributesFormatString', '%<msgName>');  OpenFcn=MessageOutputBlock
      mask Help: For detailed information please refer to the CANoe online help 'MATLAB Integration Package » CANoe I/O Library'.
      mask TypeOptions inputType: Vector | Bus Signal
      mask TypeOptions rawValue: Default | Physical value | Raw value
      mask Display:
      | image(imread('MatlabBlock.png'))
      | disp('CANoe')
  Message Output6 : Subsystem  Commented=on  AncestorBlock=canoelib/CANoe I//O/Message Output  mask(Signal Output Module){dbName=main_bus, nodeName=HPDM1, msgName=hpdm1_cooling_status4, inputType=Bus Signal, rawValue=Default}
      mask prompts: dbName "Database name"; nodeName "Node name"; msgName "Message name"; inputType "Input type"; rawValue "Raw value"
      mask help: Output module for all signals of a databasemessage provided by the CANoe interaction layer. Double click the block for configuration.
      settings: AttributesFormatString=%<msgName>  CopyFcn=set_param(gcb, 'AttributesFormatString', '%<msgName>');  OpenFcn=MessageOutputBlock
      mask Help: For detailed information please refer to the CANoe online help 'MATLAB Integration Package » CANoe I/O Library'.
      mask TypeOptions inputType: Vector | Bus Signal
      mask TypeOptions rawValue: Default | Physical value | Raw value
      mask Display:
      | image(imread('MatlabBlock.png'))
      | disp('CANoe')
  Message Output9 : Subsystem  Commented=on  AncestorBlock=canoelib/CANoe I//O/Message Output  mask(Signal Output Module){dbName=main_bus, nodeName=HPDM3, msgName=charger_data, inputType=Bus Signal, rawValue=Default}
      mask prompts: dbName "Database name"; nodeName "Node name"; msgName "Message name"; inputType "Input type"; rawValue "Raw value"
      mask help: Output module for all signals of a databasemessage provided by the CANoe interaction layer. Double click the block for configuration.
      settings: AttributesFormatString=%<msgName>  CopyFcn=set_param(gcb, 'AttributesFormatString', '%<msgName>');  OpenFcn=MessageOutputBlock
      mask Help: For detailed information please refer to the CANoe online help 'MATLAB Integration Package » CANoe I/O Library'.
      mask TypeOptions inputType: Vector | Bus Signal
      mask TypeOptions rawValue: Default | Physical value | Raw value
      mask Display:
      | image(imread('MatlabBlock.png'))
      | disp('CANoe')
  One10 : Constant  Commented=on  OutDataTypeStr=Inherit: Inherit via back propagation
  One4 : Constant  Commented=on  OutDataTypeStr=Inherit: Inherit via back propagation
  Signal Input1 : canoelib/CANoe I//O/Signal Input  Commented=on  dbName=dynamic_systems2_bus  nodeName=GVCU  msgName=pwr_steer_info_ds2  sigName=steering_wheel_angle  editSampleTime=0  rawValue=Default  dataType=Default  dataTypeDB=uint16  hasEncoding=on
      settings: AttributesFormatString=%<sigName>  SourceProductName=Vector CANoe
  Signal Output : canoelib/CANoe I//O/Signal Output  Commented=on  dbName=dynamic_systems1_bus  nodeName=GVCU  msgName=pwr_steer_ds1  sigName=steer_whl_ag  rawValue=Default  dataType=Default  dataTypeDB=uint16  hasEncoding=on
      settings: AttributesFormatString=%<sigName>  SourceProductName=Vector CANoe
  Signal Output1 : canoelib/CANoe I//O/Signal Output  Commented=on  dbName=main_bus  nodeName=SCU  msgName=scu_hmi_veh_req  sigName=drv_mod_req  rawValue=Default  dataType=Default  dataTypeDB=uint8  hasEncoding=off
      settings: AttributesFormatString=%<sigName>  SourceProductName=Vector CANoe
  Signal Output2 : canoelib/CANoe I//O/Signal Output  Commented=on  dbName=dynamic_systems1_bus  nodeName=GVCU  msgName=pwr_steer_ds1  sigName=steer_whl_snsr_v  rawValue=Default  dataType=Default  dataTypeDB=boolean  hasEncoding=off
      settings: AttributesFormatString=%<sigName>  SourceProductName=Vector CANoe
  Signal Output3 : canoelib/CANoe I//O/Signal Output  Commented=on  dbName=main_bus  nodeName=SCU  msgName=scu_hmi_veh_req  sigName=drv_cfg_req  rawValue=Default  dataType=Default  dataTypeDB=uint8  hasEncoding=off
      settings: AttributesFormatString=%<sigName>  SourceProductName=Vector CANoe
  Signal Output4 : canoelib/CANoe I//O/Signal Output  Commented=on  dbName=main_bus  nodeName=SCU  msgName=scu_hmi_veh_req  sigName=forced_chrg_btn_st  rawValue=Default  dataType=Default  dataTypeDB=uint8  hasEncoding=off
      settings: AttributesFormatString=%<sigName>  SourceProductName=Vector CANoe
  Signal Output5 : canoelib/CANoe I//O/Signal Output  Commented=on  dbName=main_bus  nodeName=SCU  msgName=scu_hmi_veh_req  sigName=esp_st_req  rawValue=Default  dataType=Default  dataTypeDB=uint8  hasEncoding=off
      settings: AttributesFormatString=%<sigName>  SourceProductName=Vector CANoe
  Signal Output6 : canoelib/CANoe I//O/Signal Output  Commented=on  dbName=dynamic_systems1_bus  nodeName=EPSA  msgName=pwr_steer_val  sigName=steer_whl_rot_spd  rawValue=Default  dataType=Default  dataTypeDB=uint16  hasEncoding=on
      settings: AttributesFormatString=%<sigName>  SourceProductName=Vector CANoe
  Switch : Switch  Commented=on  Criteria=u2 > Threshold  SaturateOnIntegerOverflow=off  InputSameDT=off
  Switch1 : Switch  Commented=on  Criteria=u2 > Threshold  SaturateOnIntegerOverflow=off  InputSameDT=off
  System Variable Input1 : canoelib/CANoe I//O/System Variable Input  Commented=on  nsName=Checker_Simulink  sysVarName=start_seq_simu  arrayIndex=-1  editSampleTime=0  rawValue=Default  dataType=Default  dataTypeDB=int32  hasEncoding=off  dataTypeCANoe=Get from CANoe
      settings: AttributesFormatString=%<nsName>::%<sysVarName>  SourceProductName=Vector CANoe
  System Variable Input3 : canoelib/CANoe I//O/System Variable Input  Commented=on  nsName=Checker_Simulink  sysVarName=start_seq_simu  arrayIndex=-1  editSampleTime=0  rawValue=Default  dataType=Default  dataTypeDB=int32  hasEncoding=off  dataTypeCANoe=Get from CANoe
      settings: AttributesFormatString=%<nsName>::%<sysVarName>  SourceProductName=Vector CANoe
  System Variable Output10 : canoelib/CANoe I//O/System Variable Output  Commented=on  nsName=Simulink_startup_variables  sysVarName=e2e_checksum_ds1  arrayIndex=-1  rawValue=Default  dataType=Default  dataTypeDB=int32  hasEncoding=off  dataTypeCANoe=Get from CANoe
      settings: AttributesFormatString=%<nsName>::%<sysVarName>  SourceProductName=Vector CANoe
  System Variable Output11 : canoelib/CANoe I//O/System Variable Output  Commented=on  nsName=Simulink_startup_variables  sysVarName=e2e_alive_counter_ds1  arrayIndex=-1  rawValue=Default  dataType=Default  dataTypeDB=int32  hasEncoding=off  dataTypeCANoe=Get from CANoe
      settings: AttributesFormatString=%<nsName>::%<sysVarName>  SourceProductName=Vector CANoe
  System Variable Output12 : canoelib/CANoe I//O/System Variable Output  Commented=on  nsName=Simulink_startup_variables  sysVarName=steer_tq_ds1  arrayIndex=-1  rawValue=Default  dataType=Default  dataTypeDB=int32  hasEncoding=off  dataTypeCANoe=Get from CANoe
      settings: AttributesFormatString=%<nsName>::%<sysVarName>  SourceProductName=Vector CANoe
  System Variable Output4 : canoelib/CANoe I//O/System Variable Output  Commented=on  nsName=VTS  sysVarName=VT7101_1_Out2::Active  arrayIndex=-1  rawValue=Default  dataType=Default  dataTypeDB=int32  hasEncoding=off  dataTypeCANoe=Get from CANoe
      settings: AttributesFormatString=%<nsName>::%<sysVarName>  SourceProductName=Vector CANoe
  System Variable Output5 : canoelib/CANoe I//O/System Variable Output  Commented=on  nsName=VTS  sysVarName=VT7101_1_Out2::AuxActive  arrayIndex=-1  rawValue=Default  dataType=Default  dataTypeDB=int32  hasEncoding=off  dataTypeCANoe=Get from CANoe
      settings: AttributesFormatString=%<nsName>::%<sysVarName>  SourceProductName=Vector CANoe
  Zero{,1..17,20..77,90..96,98..100,113..137,144..150,157..162,182} (125 alike) : Constant  Commented=on  Value=0  OutDataTypeStr=Inherit: Inherit via back propagation
  Zero{138..143,151..156} (12 alike) : Constant  Commented=on  OutDataTypeStr=Inherit: Inherit via back propagation
  Zero97 : Constant  Commented=on  Value=5  OutDataTypeStr=Inherit: Inherit via back propagation
  wires:
  Bus Creator12/1 -> Message Output12/1(In1)
  Zero161/1 -> Bus Creator16/12  "snsr_data_fr"
  Zero71/1 -> Bus Creator6/41  "hv_bat_pump_can_collision"
  Zero52/1 -> Bus Creator6/22  "front_left_fan_bat_vltg"
  Zero118/1 -> Bus Creator12/11  "e_motor_pump_speed"
  Zero157/1 -> Bus Creator16/8  "snsr_data_fll"
  Zero117/1 -> Bus Creator12/10  "hv_bat_pump_fault"
  Zero136/1 -> Bus Creator14/4  "u_wishbone_angle_fr"
  Zero159/1 -> Bus Creator16/10  "snsr_data_fcl"
  Zero155/1 -> Bus Creator16/6  "snsr_st_fr"
  Zero35/1 -> Bus Creator6/5  "front_right_fan_can_watchdog"
  Zero41/1 -> Bus Creator6/11  "center_right_fan_over_temp"
  Zero123/1 -> Bus Creator12/3  "front_left_fan_speed"
  Zero53/1 -> Bus Creator6/23  "front_left_fan_over_pwr"
  Zero147/1 -> Bus Creator15/11  "snsr_data_rcr"
  Zero135/1 -> Bus Creator14/3  "u_wishbone_angle_fl"
  Zero158/1 -> Bus Creator16/9  "snsr_data_fl"
  Zero76/1 -> Bus Creator6/46  "e_mot_pump_vltg_err"
  Zero31/1 -> Bus Creator6/1  "front_right_fan_bat_vltg"
  Zero13/1 -> Bus Creator2/9  "front_center_right_fan_warning"
  Zero154/1 -> Bus Creator16/5  "snsr_st_fl"
  Zero55/1 -> Bus Creator6/25  "front_left_fan_over_temp"
  Zero139/1 -> Bus Creator15/3  "snsr_st_rcl"
  Zero60/1 -> Bus Creator6/30  "inverter_pump_over_pwr"
  Zero119/1 -> Bus Creator12/12  "e_motor_pump_power_on"
  Bus Creator6/1 -> Message Output6/1(In1)
  Zero127/1 -> Bus Creator13/1  "e2e_checksum_disabled"
  Zero124/1 -> Bus Creator12/14  "e_motor_pump_fault"
  Zero43/1 -> Bus Creator6/13  "center_right_fan_can_collision"
  Zero21/1 -> Bus Creator4/2  "E2eChecksum"
  Zero23/1 -> Bus Creator4/4  "RearCrash"
  Zero57/1 -> Bus Creator6/27  "front_left_fan_can_collision"
  Zero68/1 -> Bus Creator6/38  "hv_bat_pump_over_crnt"
  Bus Creator5/1 -> Message Output5/1(In1)
  Zero42/1 -> Bus Creator6/12  "center_right_fan_can_watchdog"
  Zero40/1 -> Bus Creator6/10  "center_right_fan_over_crnt"
  Zero140/1 -> Bus Creator15/4  "snsr_st_rcr"
  Zero34/1 -> Bus Creator6/4  "front_right_fan_over_temp"
  Zero38/1 -> Bus Creator6/8  "center_right_fan_bat_vltg"
  Zero75/1 -> Bus Creator6/45  "e_mot_pump_over_crnt"
  Zero5/1 -> Bus Creator2/2  "e2e_alive_counter_disabled"
  Zero116/1 -> Bus Creator12/9  "hv_bat_pump_warning"
  Zero141/1 -> Bus Creator15/5  "snsr_st_rl"
  Zero66/1 -> Bus Creator6/36  "hv_bat_pump_bat_vltg"
  Zero120/1 -> Bus Creator12/13  "e_motor_pump_warning"
  Zero30/1 -> Bus Creator5/3  "CrashOutput"
  Zero20/1 -> Bus Creator4/1  "E2eAliveCounter"
  Zero74/1 -> Bus Creator6/44  "e_mot_pump_over_temp"
  Zero49/1 -> Bus Creator6/19  "center_left_fan_can_watchdog"
  Zero69/1 -> Bus Creator6/39  "hv_bat_pump_over_temp"
  Zero149/1 -> Bus Creator15/13  "snsr_data_rrl"
  Zero51/1 -> Bus Creator6/21  "center_left_fan_motor_stall"
  Zero16/1 -> Bus Creator2/12  "front_center_left_fan_power_on"
  Zero63/1 -> Bus Creator6/33  "inverter_pump_can_watchdog"
  Zero26/1 -> Bus Creator4/7  "DriverSideCrash"
  Zero4/1 -> Bus Creator2/1  "e2e_checksum_disabled"
  Zero125/1 -> Bus Creator12/4  "front_left_fan_power_on"
  Zero143/1 -> Bus Creator15/7  "snsr_st_rrl"
  Zero58/1 -> Bus Creator6/28  "front_left_fan_motor_stall"
  Zero113/1 -> Bus Creator12/6  "front_left_fan_fault"
  Zero11/1 -> Bus Creator2/7  "front_center_right_fan_speed"
  Zero138/1 -> Bus Creator15/2  "snsr_st_rll"
  Zero137/1 -> Bus Creator15/1  "actv_re"
  Zero22/1 -> Bus Creator4/3  "RolloverCrash"
  Zero48/1 -> Bus Creator6/18  "center_left_fan_over_temp"
  Zero27/1 -> Bus Creator4/8  "CrashSeverity"
  Zero148/1 -> Bus Creator15/12  "snsr_data_rr"
  Zero132/1 -> Bus Creator13/6  "inverter_pump_fault"
  Zero39/1 -> Bus Creator6/9  "center_right_fan_over_pwr"
  Bus Creator2/1 -> Message Output2/1(In1)
  Zero156/1 -> Bus Creator16/7  "snsr_st_frl"
  Zero45/1 -> Bus Creator6/15  "center_left_fan_bat_vltg"
  Zero150/1 -> Bus Creator16/1  "actv_frnt"
  Zero133/1 -> Bus Creator14/1  "u_lift_cyl_fl"
  Zero73/1 -> Bus Creator6/43  "e_mot_pump_int_op_fault"
  Zero32/1 -> Bus Creator6/2  "front_right_fan_over_pwr"
  Zero122/1 -> Bus Creator12/2  "e2e_alive_counter_disabled"
  Zero146/1 -> Bus Creator15/10  "snsr_data_rcl"
  Zero29/1 -> Bus Creator5/2  "E2eAliveCounter"
  Zero10/1 -> Bus Creator2/6  "front_right_fan_fault"
  Zero64/1 -> Bus Creator6/34  "inverter_pump_can_collision"
  Zero12/1 -> Bus Creator2/8  "front_center_right_fan_power_on"
  Zero134/1 -> Bus Creator14/2  "u_lift_cyl_fr"
  Zero7/1 -> Bus Creator2/14  "front_center_left_fan_fault"
  Zero9/1 -> Bus Creator2/5  "front_right_fan_warning"
  Zero131/1 -> Bus Creator13/5  "inverter_pump_warning"
  Zero36/1 -> Bus Creator6/6  "front_right_fan_can_collision"
  Zero114/1 -> Bus Creator12/7  "hv_bat_pump_speed"
  Zero160/1 -> Bus Creator16/11  "snsr_data_fcr"
  Bus Creator16/1 -> Message Output16/1(In1)
  Zero130/1 -> Bus Creator13/4  "inverter_pump_power_on"
  Zero28/1 -> Bus Creator5/1  "E2eChecksum"
  Zero59/1 -> Bus Creator6/29  "inverter_pump_bat_vltg"
  Zero17/1 -> Bus Creator2/13  "front_center_left_fan_warning"
  Zero151/1 -> Bus Creator16/2  "snsr_st_fll"
  Zero121/1 -> Bus Creator12/1  "e2e_checksum_disabled"
  Zero54/1 -> Bus Creator6/24  "front_left_fan_over_crnt"
  Bus Creator14/1 -> Message Output14/1(In1)
  Zero33/1 -> Bus Creator6/3  "front_right_fan_over_crnt"
  Zero24/1 -> Bus Creator4/5  "PassSideCrash"
  Zero162/1 -> Bus Creator16/13  "snsr_data_frl"
  Zero115/1 -> Bus Creator12/8  "hv_bat_pump_power_on"
  Zero144/1 -> Bus Creator15/8  "snsr_data_rll"
  Zero142/1 -> Bus Creator15/6  "snsr_st_rr"
  Zero25/1 -> Bus Creator4/6  "FrontCrash"
  Zero153/1 -> Bus Creator16/4  "snsr_st_fcr"
  Zero145/1 -> Bus Creator15/9  "snsr_data_rl"
  Zero129/1 -> Bus Creator13/3  "inverter_pump_speed"
  Zero46/1 -> Bus Creator6/16  "center_left_fan_over_pwr"
  Zero126/1 -> Bus Creator12/5  "front_left_fan_warning"
  Bus Creator15/1 -> Message Output15/1(In1)
  Zero72/1 -> Bus Creator6/42  "hv_bat_pump_motor_stall"
  Zero77/1 -> Bus Creator6/47  "e_mot_pump_comm_fault"
  Zero56/1 -> Bus Creator6/26  "front_left_fan_can_watchdog"
  Zero44/1 -> Bus Creator6/14  "center_right_fan_motor_stall"
  Zero47/1 -> Bus Creator6/17  "center_left_fan_over_crnt"
  Zero65/1 -> Bus Creator6/35  "inverter_pump_motor_stall"
  Zero152/1 -> Bus Creator16/3  "snsr_st_fcl"
  Zero62/1 -> Bus Creator6/32  "inverter_pump_over_temp"
  Zero61/1 -> Bus Creator6/31  "inverter_pump_over_crnt"
  Zero70/1 -> Bus Creator6/40  "hv_bat_pump_can_watchdog"
  Zero67/1 -> Bus Creator6/37  "hv_bat_pump_over_pwr"
  Zero8/1 -> Bus Creator2/4  "front_right_fan_power_on"
  Bus Creator13/1 -> Message Output13/1(In1)
  Zero37/1 -> Bus Creator6/7  "front_right_fan_motor_stall"
  Zero6/1 -> Bus Creator2/3  "front_right_fan_speed"
  Zero50/1 -> Bus Creator6/20  "center_left_fan_can_collision"
  Zero14/1 -> Bus Creator2/10  "front_center_right_fan_fault"
  Zero128/1 -> Bus Creator13/2  "e2e_alive_counter_disabled"
  Zero15/1 -> Bus Creator2/11  "front_center_left_fan_speed"
  Bus Creator4/1 -> Message Output4/1(In1)
  Zero2/1 -> Bus Creator20/1  "E2eChecksum_Disable"
  Constant18/1 -> Bus Creator20/8  "esp_st_req"
  Constant11/1 -> Signal Output4/1
  From6/1 -> Bus Creator20/11
  One10/1 -> Bus Creator20/10  "lift_mod_btn_st"
  Constant9/1 -> Signal Output3/1
  One4/1 -> Bus Creator20/9  "auto_upsh_btn_st"
  Zero1/1 -> Bus Creator20/2  "E2eAliveCounter_Disable"
  Zero182/1 -> Bus Creator20/13  "acc_dft_actv_st"
  Bus Creator20/1 -> Message Output20/1(In1)
  From7/1 -> Signal Output1/1
  Zero3/1 -> Bus Creator20/12  "acc_dft_dist_lvl"
  Constant16/1 -> Bus Creator20/5  "forced_chrg_btn_st"
  Constant12/1 -> Bus Creator20/4  "drv_cfg_req"
  Constant17/1 -> Bus Creator20/6  "man_mod_btn_st"
  Constant31/1 -> Bus Creator20/3  "suppg_mod_req"
  Constant10/1 -> Bus Creator20/7  "tire_mdl_req"
  Constant13/1 -> Signal Output5/1
  Zero100/1 -> Bus Creator9/11  "obc_pump_req"
  Zero98/1 -> Bus Creator9/9  "evcc_status"
  Zero92/1 -> Bus Creator9/3  "charging_mode"
  Zero96/1 -> Bus Creator9/7  "inlet_motor_status"
  Zero95/1 -> Bus Creator9/6  "charge_voltage"
  Bus Creator9/1 -> Message Output9/1(In1)
  Zero93/1 -> Bus Creator9/4  "charge_port_status"
  Zero94/1 -> Bus Creator9/5  "charge_current"
  Zero90/1 -> Bus Creator9/1  "e2e_checksum_disabled"
  Zero99/1 -> Bus Creator9/10  "obc_fan_req"
  Zero91/1 -> Bus Creator9/2  "e2e_alive_counter_disabled"
  Zero97/1 -> Bus Creator9/8  "obc_status"
  Constant8/1 -> Switch1/3
  Switch1/1 -> System Variable Output5/1
  Signal Input1/1 -> Display2/1
  Switch/1 -> System Variable Output4/1
  Constant4/1 -> System Variable Output10/1  "e2e_checksum"
  System Variable Input1/1 -> Switch1/2
  Constant5/1 -> System Variable Output11/1  "e2e_alive_counter"
  Constant7/1 -> Switch/1
  System Variable Input3/1 -> Switch/2
  Constant1/1 -> Signal Output2/1  "steer_whl_snsr_v"
  Zero/1 -> Switch/3
  Constant3/1 -> Signal Output/1  "steer_whl_ag"
  Constant6/1 -> System Variable Output12/1  "steer_tq"
  Constant2/1 -> Signal Output6/1  "steer_whl_rot_spd"
  Constant14/1 -> Switch1/1

== system GVCU_HIL/GVCU - HiL/Message Output1 ==
  In1 : Inport
  Bus Selector : BusSelector  OutputSignals=pack_current,pack_voltage
  S-Function_1 : S-Function  FunctionName=sigout  Parameters=dbName;nodeName;msgName;2;'pack_current';'pack_voltage';VGetRawValueFlag(rawValue);'inherited'  SFunctionDeploymentMode=off  EnableBusSupport=off
      settings: AttributesFormatString=pack_current\npack_voltage\n
  wires:
  In1/1 -> Bus Selector/1
  Bus Selector/1 -> S-Function_1/1  "<pack_current>"
  Bus Selector/2 -> S-Function_1/2  "<pack_voltage>"
